simulink model "HIL5DOF_Speedgoat"  (R2026a)
settings: Solver=ode3  StopTime=inf  FixedStep=1/20000
values from neighbouring files (symbols this model uses):
  ems =     [ems11.mat]
  hems =     [Datos_Para_Control_Preciso.mat]
undefined symbols (not defined in the file or in its folder): hems_direct_F_table_H10, hems_direct_gap_bp_H10, hems_direct_I_bp_H10, IO316, IO3xx, m, magnitude, Pull, pull, up, x0, xguid_12, xguid_34, xguid_56, xlev_12, xlev_34, ylev_13, ylev_24, zguid
libraries: speedgoatlib_IO110 x2, aerolibobsolete x1, speedgoatlib_fpga_pwm x1, speedgoatlib_fpga x1
(part 1 of 2)
settings Model: Creator=Mutti  LastModifiedBy=Mutti
settings SolverCC: ConcurrentTasks=on  PositivePriorityOrder=on
settings OptimizationCC: OptimizeBlockIOStorage=off
settings DebuggingCC: TasksWithSamePriorityMsg=none
settings HardwareCC: ProdBitPerLong=64.0  ProdHWDeviceType=Intel->x86-64 (Linux 64)
settings RTWCC: SystemTargetFile=speedgoat.tlc  TemplateMakefile=slrealtime_default_tmf  Toolchain=Simulink Real-Time Toolchain  BuildConfiguration=Faster Runs  TargetLang=C++  Description=Speedgoat Real-Time Target Machine
settings SimulinkRealTimeTargetCC: SLRTFileLogMaxRuns=1.0  TargetLangStandard=C++11 (ISO)  MultiwordLength=2048.0  MATLABClassNameForMDSCustomization=Simulink.SoftwareTarget.GRTCustomization

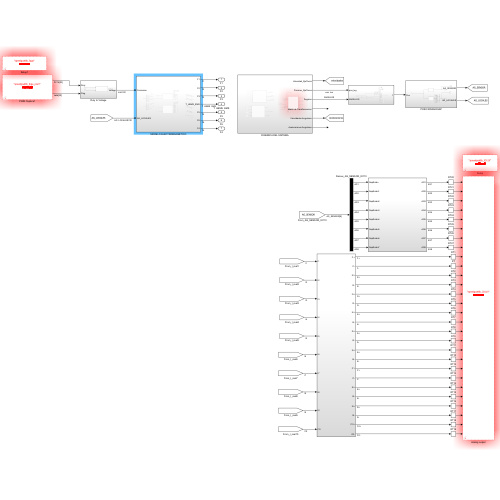
[thumbnail: Simulink's stored preview of the top-level diagram]
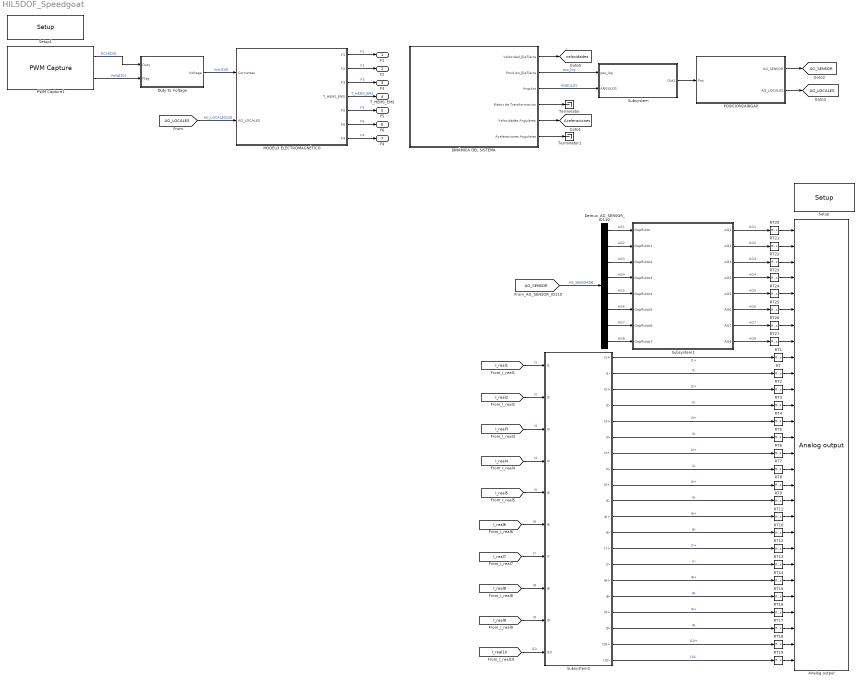
== system HIL5DOF_Speedgoat ==
  Analog output : speedgoatlib_IO110/Analog output  id=1  ts=1/2000  channels=[1,2,3,4,5,6,7,8,9,10,11,12,13,14,15,16,17,18,19,20,21,22,23,24,25,26,27,28]  range=[4,4,4,4,4,4,4,4,4,4,4,4,4,4,4,4,4,4,4,4,4,4,4,4,4,4,4,4,4,4,4,4]  pciSlot=-1  init=[0,0,0,0,0,0,0,0,0,0,0,0,0,0,0,0,0,0,0,0,0,0,0,0,0,0,0,0]  reset=[1,1,1,1,1,1,1,1,1,1,1,1,1,1,1,1,1,1,1,1,1,1,1,1,1,1,1,1]
      settings: SourceProductName=IO110
  DINÁMICA DEL SISTEMA : Subsystem
  Demux_AG_SENSOR_IO110 : Demux  Outputs=8
  Duty to Voltage : Subsystem
  MODELO ELECTROMAGNÉTICO : Subsystem
  POSICION2AIRGAP : Subsystem
  PWM Capture1 : speedgoatlib_fpga_pwm/PWM Capture  id=1  chan=[1:20]  ts=1/1000  captureMode=High transitions triggered  bit_width_cap=24  captureTimeout_si=0.5e-3  captureTimeout_eff=[500e-6]  debounce_si=10e-6  debounce_eff=[10e-6]  showHighDuration=off  showLowDuration=off  showPeriod=off  showDC16=on  showDC8=off  showTOn=off  showTOff=off  showValidData=on
      settings: SourceProductName=PWM
  RT{,1..19} (20 alike) : RateTransition  OutPortSampleTime=5e-05
  RT{20..27} (8 alike) : RateTransition  OutPortSampleTime=1/7500
  Setup : speedgoatlib_IO110/Setup  group=Module setup  id=1  daChannel=[1:28]  daInitValue=zeros(1,28)  daReset=[1]  pciSlot=-1  daRange00=-10V .. +10V  daRange01=-10V .. +10V  daRange02=-10V .. +10V  daRange03=-10V .. +10V  daTSD0=off  daClamp0=on  daRange10=-10V .. +10V  daRange11=-10V .. +10V  daRange12=-10V .. +10V  daRange13=-10V .. +10V  daTSD1=off  daClamp1=on  daRange20=-10V .. +10V  daRange21=-10V .. +10V  daRange22=-10V .. +10V  daRange23=-10V .. +10V  daTSD2=off  daClamp2=on  daRange30=-10V .. +10V  daRange31=-10V .. +10V  daRange32=-10V .. +10V  daRange33=-10V .. +10V  daTSD3=off  daClamp3=on  daRange40=-10V .. +10V  daRange41=-10V .. +10V  daRange42=-10V .. +10V  daRange43=-10V .. +10V  daTSD4=off  daClamp4=on  daRange50=-10V .. +10V  daRange51=-10V .. +10V  daRange52=-10V .. +10V  daRange53=-10V .. +10V  daTSD5=off  daClamp5=on  daRange60=-10V .. +10V  daRange61=-10V .. +10V  daRange62=-10V .. +10V  daRange63=-10V .. +10V  daTSD6=off  daClamp6=on  daRange70=-10V .. +10V  daRange71=-10V .. +10V  daRange72=-10V .. +10V  daRange73=-10V .. +10V  daTSD7=off  daClamp7=on
      settings: SourceProductName=IO110
  Setup1 : speedgoatlib_fpga/Setup/Setup  board=IO316-100k  id=1  pciSlot=-1  device_id=1  bitstreamFilePath=C:\Users\Mutti\Documents\Hyperloop\SpeedGoat\speedgoat_IO316_100k_21_CI_02826_v2\  bitstreamFile=speedgoat_IO316_100k_21_CI_02826_v2.mat  fpgaFreq=[75000000 100000000]  enableDma=off  rearEnb_1=on  rearIO_1=IO3xx-21  rearEnb_2=off  rearIO_2=None  ProgSpiFlash=off  ProgBPIFlash=off  useFpgaDmaController=off  dmaTrigDropdown=Model Step  dmaTrigSelect=0  dmaStopOnOverload=on  dmaModeSequential=on  dmaModeParallel=off  PullRPort15=pull-up 3.3V  PullRPort31=pull-up 3.3V  PullRPort47=pull-up 3.3V  PullRPort63=pull-up 3.3V  diffLineTermination_1=on  diffLineTermination_2=on  diffLineTermination_3=on  diffLineTermination_4=on  diffLineTermination_5=on  diffLineTermination_6=on  diffLineTermination_7=on  diffLineTermination_8=on  diffLineTermination_9=on  diffLineTermination_10=on  diffLineTermination_11=on  diffLineTermination_12=on  diffLineTermination_13=on  diffLineTermination_14=on  diffLineTermination_15=on  diffLineTermination_16=on  diffLineTermination_17=on  diffLineTermination_18=on  diffLineTermination_19=on  diffLineTermination_20=on  diffLineTermination_21=on  diffLineTermination_22=on  diffLineTermination_23=on  diffLineTermination_24=on  diffLineTermination_25=on  diffLineTermination_26=on  diffLineTermination_27=on  diffLineTermination_28=on  diffLineTermination_29=on  diffLineTermination_30=on  diffLineTermination_31=on  diffLineTermination_32=on  ioVoltageDropDown1=3.3V  pullResistorDropDown1_1=Pull-up  pullResistorDropDown1_2=Pull-up  pullResistorDropDown1_3=Pull-up  pullResistorDropDown1_4=Pull-up  pullResistorDropDown1_5=Pull-up  pullResistorDropDown1_6=Pull-up  pullResistorDropDown1_7=Pull-up  pullResistorDropDown1_8=Pull-up  ttlIsImplementedCheckBox1=off  pullResistorDropDown2=Pull-up  ioVoltageDropDown2=3.3V  ttlIsImplementedCheckBox2=off  pullResistorDropDown3=Pull-up  ioVoltageDropDown3=3.3V  ttlIsImplementedCheckBox3=off  pullResistorDropDown4=Pull-up  ioVoltageDropDown4=3.3V  ttlIsImplementedCheckBox4=off  pullResistorDropDown5=Pull-up  ioVoltageDropDown5=3.3V  ttlIsImplementedCheckBox5=off  pullResistorDropDown6=Pull-up  ioVoltageDropDown6=3.3V  ttlIsImplementedCheckBox6=off  pullResistorDropDown7=Pull-up  ioVoltageDropDown7=3.3V  ttlIsImplementedCheckBox7=off  pullResistorDropDown8=Pull-up  ioVoltageDropDown8=3.3V  ttlIsImplementedCheckBox8=off  terminationCheckBox1=off  terminationCheckBox2=off  terminationCheckBox3=off  terminationCheckBox4=off  diffIsImplementedCheckBox1=off  terminationCheckBox5=off  terminationCheckBox6=off  terminationCheckBox7=off  terminationCheckBox8=off  diffIsImplementedCheckBox2=off  terminationCheckBox9=off  terminationCheckBox10=off  terminationCheckBox11=off  terminationCheckBox12=off  diffIsImplementedCheckBox3=off  terminationCheckBox13=off  terminationCheckBox14=off  terminationCheckBox15=off  terminationCheckBox16=off  diffIsImplementedCheckBox4=off  terminationCheckBox17=off  terminationCheckBox18=off  terminationCheckBox19=off  terminationCheckBox20=off  diffIsImplementedCheckBox5=off  terminationCheckBox21=off  terminationCheckBox22=off  terminationCheckBox23=off  terminationCheckBox24=off  diffIsImplementedCheckBox6=off  terminationCheckBox25=off  terminationCheckBox26=off  terminationCheckBox27=off  terminationCheckBox28=off  diffIsImplementedCheckBox7=off  terminationCheckBox29=off  terminationCheckBox30=off  terminationCheckBox31=off  terminationCheckBox32=off  diffIsImplementedCheckBox8=off  PullRPort0_1=pull-up  VioPort0_1=3.3V  PullRPort1_1=pull-up  VioPort1_1=3.3V  PullRPort2_1=pull-up  VioPort2_1=3.3V  PullRPort3_1=pull-up  VioPort3_1=3.3V  PullRPort4_1=pull-up  VioPort4_1=3.3V  PullRPort5_1=pull-up  VioPort5_1=3.3V  PullRPort6_1=pull-up  VioPort6_1=3.3V  diffLineTermination_rear1_1=on  diffLineTermination_rear1_2=on  diffLineTermination_rear1_3=on  diffLineTermination_rear1_4=on  diffLineTermination_rear1_5=on  diffLineTermination_rear1_6=on  diffLineTermination_rear1_7=on  diffLineTermination_rear1_8=on  PullRPort0_2=pull-up  VioPort0_2=3.3V  PullRPort1_2=pull-up  VioPort1_2=3.3V  PullRPort2_2=pull-up  VioPort2_2=3.3V  PullRPort3_2=pull-up  VioPort3_2=3.3V  PullRPort4_2=pull-up  VioPort4_2=3.3V  PullRPort5_2=pull-up  VioPort5_2=3.3V  PullRPort6_2=pull-up  VioPort6_2=3.3V  diffLineTermination_rear2_1=on  diffLineTermination_rear2_2=on  diffLineTermination_rear2_3=on  diffLineTermination_rear2_4=on  diffLineTermination_rear2_5=on  diffLineTermination_rear2_6=on  diffLineTermination_rear2_7=on  diffLineTermination_rear2_8=on
      settings: SourceProductName=IO3xx
  Subsystem : Subsystem
  Subsystem1 : Subsystem
  Subsystem2 : Subsystem
  Terminator : Terminator
  Terminator1 : Terminator
  F1 : Outport
  F2 : Outport  Port=2
  F3 : Outport  Port=3
  T_HEMS_EMS : Outport  Port=4
  F5 : Outport  Port=5
  F6 : Outport  Port=6
  F4 : Outport  Port=7
  tag scope: AG_LOCALES=global, AG_SENSOR=global, Aceleraciones=global, velocidades=global
  wires:
  POSICION2AIRGAP/1(AG_SENSOR) -> [AG_SENSOR]
  POSICION2AIRGAP/2(AG_LOCALES) -> [AG_LOCALES]
  DINÁMICA DEL SISTEMA/4(Matriz de Transformacion) -> Terminator/1
  DINÁMICA DEL SISTEMA/6(Aceleraciones Angulares) -> Terminator1/1
  DINÁMICA DEL SISTEMA/1(Velocidad_EjeTierra) -> [velocidades]
  DINÁMICA DEL SISTEMA/5(Velocidades Angulares) -> [Aceleraciones]
  PWM Capture1/1 -> Duty to Voltage/1(Duty)  "DC16[20]"
  PWM Capture1/2 -> Duty to Voltage/2(Flag)  "Valid[20]"
  Duty to Voltage/1(Voltage) -> MODELO ELECTROMAGNÉTICO/1(Corrientes)  "Vctrl[10]"
  [AG_SENSOR] -> Demux_AG_SENSOR_IO110/1  "AG_SENSOR[8]"
  Demux_AG_SENSOR_IO110/1 -> Subsystem1/1(GapRuido)  "AG1"
  Subsystem1/1(AG1) -> RT20/1  "AG1"
  Demux_AG_SENSOR_IO110/2 -> Subsystem1/2(GapRuido1)  "AG2"
  Subsystem1/2(AG2) -> RT21/1  "AG2"
  Demux_AG_SENSOR_IO110/3 -> Subsystem1/3(GapRuido2)  "AG3"
  Subsystem1/3(AG3) -> RT22/1  "AG3"
  Demux_AG_SENSOR_IO110/4 -> Subsystem1/4(GapRuido3)  "AG4"
  Subsystem1/4(AG4) -> RT23/1  "AG4"
  Demux_AG_SENSOR_IO110/5 -> Subsystem1/5(GapRuido4)  "AG5"
  Subsystem1/5(AG5) -> RT24/1  "AG5"
  Demux_AG_SENSOR_IO110/6 -> Subsystem1/6(GapRuido5)  "AG6"
  Subsystem1/6(AG6) -> RT25/1  "AG6"
  Demux_AG_SENSOR_IO110/7 -> Subsystem1/7(GapRuido6)  "AG7"
  Subsystem1/7(AG7) -> RT26/1  "AG7"
  Demux_AG_SENSOR_IO110/8 -> Subsystem1/8(GapRuido7)  "AG8"
  Subsystem1/8(AG8) -> RT27/1  "AG8"
  [I_real1] -> Subsystem2/1(I1)  "I1"
  [I_real2] -> Subsystem2/2(I2)  "I2"
  [I_real3] -> Subsystem2/3(I3)  "I3"
  [I_real4] -> Subsystem2/4(I4)  "I4"
  [I_real5] -> Subsystem2/5(I5)  "I5"
  [I_real6] -> Subsystem2/6(I6)  "I6"
  [I_real7] -> Subsystem2/7(I7)  "I7"
  [I_real8] -> Subsystem2/8(I8)  "I8"
  [I_real9] -> Subsystem2/9(I9)  "I9"
  [I_real10] -> Subsystem2/10(I10)  "I10"
  Subsystem2/1(I1+) -> RT1/1  "I1+"
  Subsystem2/2(I1-) -> RT/1  "I1-"
  Subsystem2/3(I2+) -> RT2/1  "I2+"
  Subsystem2/4(I2-) -> RT3/1  "I2-"
  Subsystem2/5(I3+) -> RT4/1  "I3+"
  Subsystem2/6(I3-) -> RT5/1  "I3-"
  Subsystem2/7(I4+) -> RT6/1  "I4+"
  Subsystem2/8(I4-) -> RT7/1  "I4-"
  Subsystem2/9(I5+) -> RT8/1  "I5+"
  Subsystem2/10(I5-) -> RT9/1  "I5-"
  Subsystem2/11(I6+) -> RT11/1  "I6+"
  Subsystem2/12(I6-) -> RT10/1  "I6-"
  Subsystem2/13(I7+) -> RT12/1  "I7+"
  Subsystem2/14(I7-) -> RT13/1  "I7-"
  Subsystem2/15(I8+) -> RT14/1  "I8+"
  Subsystem2/16(I8-) -> RT15/1  "I8-"
  Subsystem2/17(I9+) -> RT16/1  "I9+"
  Subsystem2/18(I9-) -> RT17/1  "I9-"
  Subsystem2/19(I10+) -> RT18/1  "I10+"
  Subsystem2/20(I10-) -> RT19/1  "I10-"
  [AG_LOCALES] -> MODELO ELECTROMAGNÉTICO/2(AG_LOCALES)  "AG_LOCALES[10]"
  MODELO ELECTROMAGNÉTICO/1(F1) -> F1/1  "F1"
  MODELO ELECTROMAGNÉTICO/2(F2) -> F2/1  "F2"
  MODELO ELECTROMAGNÉTICO/3(F3) -> F3/1  "F3"
  MODELO ELECTROMAGNÉTICO/4(T_HEMS_EMS) -> T_HEMS_EMS/1  "T_HEMS_EMS"
  MODELO ELECTROMAGNÉTICO/5(F5) -> F5/1  "F5"
  MODELO ELECTROMAGNÉTICO/6(F6) -> F6/1  "F6"
  MODELO ELECTROMAGNÉTICO/7(F4) -> F4/1  "F4"
  RT/1 -> Analog output/10
  RT1/1 -> Analog output/9
  RT2/1 -> Analog output/11
  RT3/1 -> Analog output/12
  RT4/1 -> Analog output/13
  RT5/1 -> Analog output/14
  RT11/1 -> Analog output/19
  RT6/1 -> Analog output/15
  RT7/1 -> Analog output/16
  RT8/1 -> Analog output/17
  RT9/1 -> Analog output/18
  RT10/1 -> Analog output/20
  RT12/1 -> Analog output/21
  RT13/1 -> Analog output/22
  RT14/1 -> Analog output/23
  RT15/1 -> Analog output/24
  RT16/1 -> Analog output/25
  RT17/1 -> Analog output/26
  RT18/1 -> Analog output/27
  RT19/1 -> Analog output/28
  RT20/1 -> Analog output/1
  RT21/1 -> Analog output/2
  RT22/1 -> Analog output/3
  RT23/1 -> Analog output/4
  RT24/1 -> Analog output/5
  RT25/1 -> Analog output/6
  RT26/1 -> Analog output/7
  RT27/1 -> Analog output/8
  DINÁMICA DEL SISTEMA/2(Posicion_EjeTierra) -> Subsystem/1(pos_log)  "pos_log"
  DINÁMICA DEL SISTEMA/3(Ángulos) -> Subsystem/2(ANGULOS)  "ANGULOS"
  Subsystem/1(Out1) -> POSICION2AIRGAP/1(Pos)

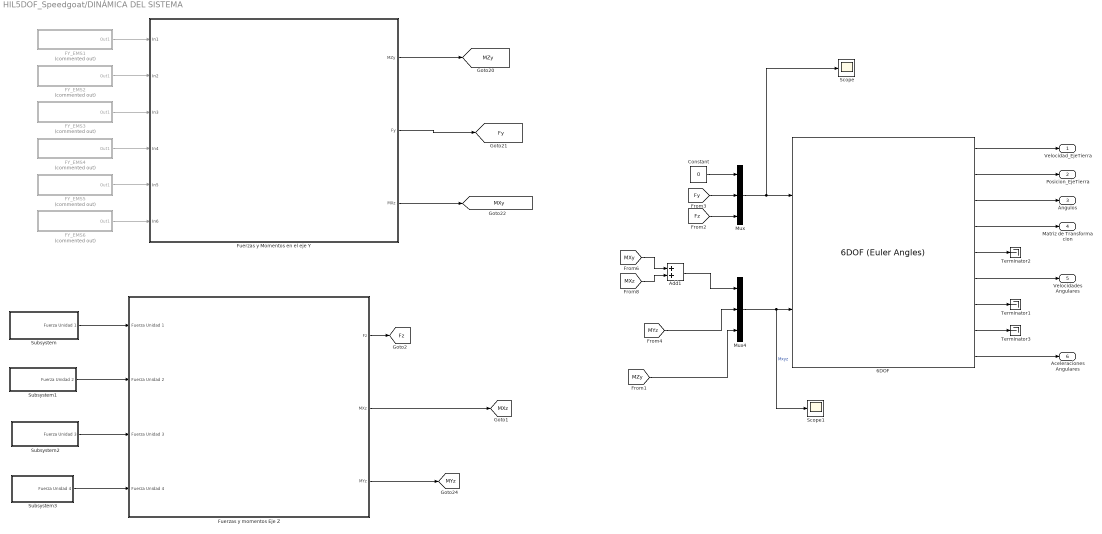
== system HIL5DOF_Speedgoat/DINÁMICA DEL SISTEMA ==
  "6DOF " : aerolibobsolete/6DOF (Euler Angles)  units=Metric (MKS)  mtype=Fixed  rep=Euler Angles  xme_0=[x0 0.000 0.025]  Vm_0=[0 0 0]  eul_0=[0 0 0]  pm_0=[0 0 0]  mass_0=m  mass_e=0.5  mass_f=2.0  inertia=I  inertia_e=eye(3)  inertia_f=2*eye(3)  k_quat=1.0  vre_flag=on  abi_flag=on  aMode=0  xme_statename=''  Vm_statename=''  eul_statename=''  quat_statename=''  pm_statename=''  mass_statename=''
  Add1 : Sum
  Constant : Constant  Value=0
  FY_EMS1 : Subsystem  Commented=on
  FY_EMS2 : Subsystem  Commented=on
  FY_EMS3 : Subsystem  Commented=on
  FY_EMS4 : Subsystem  Commented=on
  FY_EMS5 : Subsystem  Commented=on
  FY_EMS6 : Subsystem  Commented=on
  Fuerzas y Momentos en el eje Y : Subsystem
  Fuerzas y momentos Eje Z : Subsystem
  Mux : Mux  Inputs=3
  Mux4 : Mux  Inputs=3
  Scope : Scope
      settings: ActiveDisplayYMinimum=-6.71767895083E+6  ActiveDisplayYMaximum=4.200096969295E+7
  Scope1 : Scope
      settings: ActiveDisplayYMinimum=-1  ActiveDisplayYMaximum=1  DataLoggingVariableName=ScopeData2
  Subsystem : Subsystem
  Subsystem1 : Subsystem
  Subsystem2 : Subsystem
  Subsystem3 : Subsystem
  Terminator1 : Terminator
  Terminator2 : Terminator
  Terminator3 : Terminator
  Velocidad_EjeTierra : Outport
  Posicion_EjeTierra : Outport  Port=2
  Ángulos : Outport  Port=3
  Matriz de Transformacion : Outport  Port=4
  Velocidades Angulares : Outport  Port=5
  Aceleraciones Angulares : Outport  Port=6
  tag scope: Fy=global, Fz=global, MXy=global, MXz=global, MYz=global, MZy=global
  wires:
  "6DOF "/8 -> Terminator3/1
  "6DOF "/1 -> Velocidad_EjeTierra/1
  "6DOF "/5 -> Terminator2/1
  "6DOF "/4 -> Matriz de Transformacion/1
  "6DOF "/2 -> Posicion_EjeTierra/1
  "6DOF "/3 -> Ángulos/1
  "6DOF "/7 -> Terminator1/1
  "6DOF "/6 -> Velocidades Angulares/1
  [Fy] -> Mux/2
  Mux/1 -> Scope/1, "6DOF "/1
  [Fz] -> Mux/3
  Mux4/1 -> Scope1/1, "6DOF "/2  "Mxyz"
  Constant/1 -> Mux/1
  "6DOF "/9 -> Aceleraciones Angulares/1
  [MZy] -> Mux4/3
  [MXz] -> Add1/2
  [MXy] -> Add1/1
  Fuerzas y momentos Eje Z/1(Fz) -> [Fz]
  Add1/1 -> Mux4/1
  [MYz] -> Mux4/2
  Fuerzas y Momentos en el eje Y/2(Fy) -> [Fy]
  Fuerzas y momentos Eje Z/2(MXz) -> [MXz]
  Fuerzas y momentos Eje Z/3(MYz) -> [MYz]
  Fuerzas y Momentos en el eje Y/3(MXz) -> [MXy]
  Fuerzas y Momentos en el eje Y/1(MZy) -> [MZy]
  FY_EMS1/1(Out1) -> Fuerzas y Momentos en el eje Y/1(In1)
  FY_EMS6/1(Out1) -> Fuerzas y Momentos en el eje Y/6(In6)
  FY_EMS5/1(Out1) -> Fuerzas y Momentos en el eje Y/5(In5)
  FY_EMS4/1(Out1) -> Fuerzas y Momentos en el eje Y/4(In4)
  FY_EMS3/1(Out1) -> Fuerzas y Momentos en el eje Y/3(In3)
  FY_EMS2/1(Out1) -> Fuerzas y Momentos en el eje Y/2(In2)
  Subsystem3/1(Fuerza Unidad 4) -> Fuerzas y momentos Eje Z/4(Fuerza Unidad 4)
  Subsystem/1(Fuerza Unidad 1) -> Fuerzas y momentos Eje Z/1(Fuerza Unidad 1)
  Subsystem1/1(Fuerza Unidad 2) -> Fuerzas y momentos Eje Z/2(Fuerza Unidad 2)
  Subsystem2/1(Fuerza Unidad 3) -> Fuerzas y momentos Eje Z/3(Fuerza Unidad 3)

== system HIL5DOF_Speedgoat/Duty to Voltage ==
  Duty : Inport
  Flag : Inport  Port=2
  PWM pairs to Vctrl : MATLAB Function  TreatAsAtomicUnit=on
  Voltage : Outport
  wires:
  Duty/1 -> PWM pairs to Vctrl/1(Duty)
  Flag/1 -> PWM pairs to Vctrl/2(Flag)
  PWM pairs to Vctrl/1(Voltage) -> Voltage/1

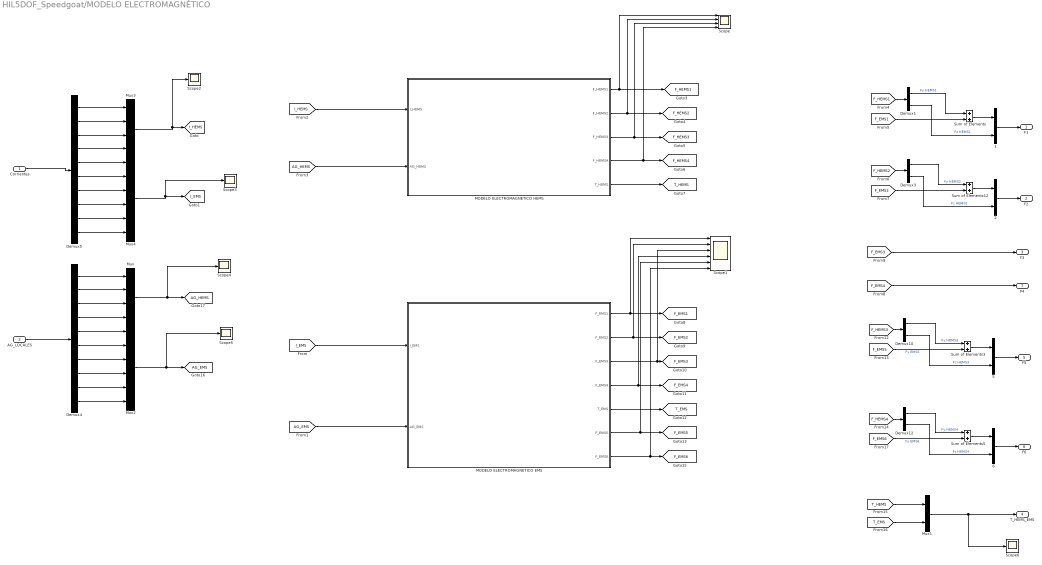
== system HIL5DOF_Speedgoat/MODELO ELECTROMAGNÉTICO ==
  Corrientes : Inport
  AG_LOCALES : Inport  Port=2
  {1..2,5..6} (4 alike) : Mux  Inputs=2
  Demux{1,3,10,12} (4 alike) : Demux  Outputs=2
  Demux4 : Demux  Outputs=10
  Demux5 : Demux  Outputs=10
  MODELO ELECTROMAGNETICO EMS : Subsystem
  MODELO ELECTROMAGNETICO HEMS : Subsystem
  Mux : Mux
  Mux1 : Mux  Inputs=2
  Mux2 : Mux  Inputs=6
  Mux3 : Mux
  Mux4 : Mux  Inputs=6
  Scope : Scope  NumInputPorts=4
      settings: ActiveDisplayYMinimum=225.21547346710162  ActiveDisplayYMaximum=548.6247825703233
  Scope1 : Scope  NumInputPorts=6
      settings: ActiveDisplayYMinimum=-3.137221535142E+7  ActiveDisplayYMaximum=2.1564141928831E+8  DataLoggingVariableName=ScopeData2
  Scope{2..6} (5 alike) : Scope
      Scope2 settings: ActiveDisplayYMinimum=-16.47415  ActiveDisplayYMaximum=23.87015
      Scope3 settings: ActiveDisplayYMinimum=-6.2499999999999982  ActiveDisplayYMaximum=56.25  DataLoggingVariableName=ScopeData2
      Scope4 settings: DataLoggingVariableName=ScopeData3
      Scope5 settings: DataLoggingVariableName=ScopeData4
      Scope6 settings: ActiveDisplayYMinimum=39.93449  ActiveDisplayYMaximum=40.58956  DataLoggingVariableName=ScopeData2
  Sum of Elements{,3,5,12} (4 alike) : Sum
  F1 : Outport
  F2 : Outport  Port=2
  F3 : Outport  Port=3
  T_HEMS_EMS : Outport  Port=4
  F5 : Outport  Port=5
  F6 : Outport  Port=6
  F4 : Outport  Port=7
  tag scope: AG_EMS=global, AG_HEMS=global, F_EMS1=global, F_EMS2=global, F_EMS3=global, F_EMS4=global, F_EMS5=global, F_EMS6=global, F_HEMS1=global, F_HEMS2=global, F_HEMS3=global, F_HEMS4=global, I_EMS=global, I_HEMS=global, T_EMS=global, T_HEMS=global
  wires:
  [I_HEMS] -> MODELO ELECTROMAGNETICO HEMS/1(I_HEMS)
  MODELO ELECTROMAGNETICO HEMS/3(F_HEMS3) -> Scope/3, [F_HEMS3]
  MODELO ELECTROMAGNETICO EMS/5(T_EMS) -> [T_EMS]
  [F_EMS2] -> Sum of Elements12/2
  [F_EMS6] -> Sum of Elements5/2  "Fy EMS6"
  MODELO ELECTROMAGNETICO EMS/3(F_EMS3) -> Scope1/3, [F_EMS3]
  MODELO ELECTROMAGNETICO EMS/6(F_EMS5) -> Scope1/5, [F_EMS5]
  MODELO ELECTROMAGNETICO EMS/1(F_EMS1) -> Scope1/1, [F_EMS1]
  [AG_HEMS] -> MODELO ELECTROMAGNETICO HEMS/2(AG_HEMS)
  Demux12/2 -> 6/2  "Fz HEMS4"
  [I_EMS] -> MODELO ELECTROMAGNETICO EMS/1(I_EMS)
  MODELO ELECTROMAGNETICO HEMS/1(F_HEMS1) -> Scope/1, [F_HEMS1]
  [F_EMS4] -> F4/1
  2/1 -> F2/1
  Demux3/2 -> 2/2  "Fz HEMS2"
  MODELO ELECTROMAGNETICO HEMS/4(F_HEMS4) -> Scope/4, [F_HEMS4]
  MODELO ELECTROMAGNETICO EMS/7(F_EMS6) -> Scope1/6, [F_EMS6]
  Demux1/2 -> 1/2  "Fz HEMS1"
  [T_HEMS] -> Mux1/1
  Sum of Elements/1 -> 1/1
  MODELO ELECTROMAGNETICO HEMS/2(F_HEMS2) -> Scope/2, [F_HEMS2]
  [F_HEMS4] -> Demux12/1
  Sum of Elements12/1 -> 2/1
  5/1 -> F5/1
  [T_EMS] -> Mux1/2
  [F_EMS1] -> Sum of Elements/2
  [F_HEMS2] -> Demux3/1
  Sum of Elements5/1 -> 6/1
  Mux1/1 -> Scope6/1, T_HEMS_EMS/1
  1/1 -> F1/1
  MODELO ELECTROMAGNETICO HEMS/5(T_HEMS) -> [T_HEMS]
  Sum of Elements3/1 -> 5/1
  [F_EMS3] -> F3/1
  [F_HEMS1] -> Demux1/1
  Demux12/1 -> Sum of Elements5/1  "Fy HEMS4"
  [F_EMS5] -> Sum of Elements3/2  "Fy EMS5"
  [F_HEMS3] -> Demux10/1
  [AG_EMS] -> MODELO ELECTROMAGNETICO EMS/2(AG_EMS)
  Demux10/2 -> 5/2  "Fz HEMS3"
  MODELO ELECTROMAGNETICO EMS/4(F_EMS4) -> Scope1/4, [F_EMS4]
  MODELO ELECTROMAGNETICO EMS/2(F_EMS2) -> Scope1/2, [F_EMS2]
  6/1 -> F6/1
  Demux1/1 -> Sum of Elements/1  "Fy HEMS1"
  Demux3/1 -> Sum of Elements12/1  "Fy HEMS2"
  Demux10/1 -> Sum of Elements3/1  "Fy HEMS3"
  AG_LOCALES/1 -> Demux4/1
  Demux4/1 -> Mux/1
  Demux4/2 -> Mux/2
  Demux4/3 -> Mux/3
  Demux4/4 -> Mux/4
  Mux/1 -> Scope4/1, [AG_HEMS]
  Mux2/1 -> Scope5/1, [AG_EMS]
  Demux4/5 -> Mux2/1
  Demux4/10 -> Mux2/6
  Demux4/9 -> Mux2/5
  Demux4/8 -> Mux2/4
  Demux4/7 -> Mux2/3
  Demux4/6 -> Mux2/2
  Demux5/6 -> Mux4/2
  Demux5/7 -> Mux4/3
  Demux5/8 -> Mux4/4
  Demux5/9 -> Mux4/5
  Demux5/10 -> Mux4/6
  Demux5/5 -> Mux4/1
  Mux4/1 -> Scope3/1, [I_EMS]
  Mux3/1 -> Scope2/1, [I_HEMS]
  Demux5/4 -> Mux3/4
  Demux5/3 -> Mux3/3
  Demux5/2 -> Mux3/2
  Demux5/1 -> Mux3/1
  Corrientes/1 -> Demux5/1

== system HIL5DOF_Speedgoat/POSICION2AIRGAP ==
  Pos : Inport
  Demux8 : Demux  Outputs=10
  Mux5 : Mux  Inputs=6
  Mux6 : Mux
  Mux7 : Mux  Inputs=2
  Pos2Airgap_AG_LOCALES : Subsystem
  Pos2Airgap_SENSOR : Subsystem
  Scope1 : Scope
      settings: ActiveDisplayYMinimum=0.0027172435687609548  ActiveDisplayYMaximum=0.025639307881151412  DataLoggingVariableName=ScopeData10
  Scope3 : Scope
      settings: ActiveDisplayYMinimum=-0.049037976197916368  ActiveDisplayYMaximum=0.44139914576247047  DataLoggingVariableName=ScopeData9
  AG_SENSOR : Outport
  AG_LOCALES : Outport  Port=2
  wires:
  Pos2Airgap_SENSOR/1(y) -> Scope3/1, AG_SENSOR/1
  Demux8/8 -> Mux5/4
  Pos2Airgap_AG_LOCALES/1(y) -> Demux8/1
  Demux8/7 -> Mux5/3
  Pos/1 -> Pos2Airgap_SENSOR/1(Pos), Pos2Airgap_AG_LOCALES/1(Pos)
  Mux6/1 -> Mux7/1
  Demux8/9 -> Mux5/5
  Demux8/6 -> Mux5/2
  Mux5/1 -> Mux7/2
  Demux8/3 -> Mux6/3
  Mux7/1 -> Scope1/1, AG_LOCALES/1
  Demux8/4 -> Mux6/4
  Demux8/2 -> Mux6/2
  Demux8/1 -> Mux6/1
  Demux8/10 -> Mux5/6
  Demux8/5 -> Mux5/1

== system HIL5DOF_Speedgoat/Subsystem ==
  pos_log : Inport
  ANGULOS : Inport  Port=2
  Demux : Demux  Outputs=3
  Demux1 : Demux  Outputs=3
  Mux : Mux  Inputs=5
  Mux2 : Mux  Inputs=3
  Saturation1 : Saturate  UpperLimit=0.2  LowerLimit=-0.2
  Saturation2 : Saturate  UpperLimit=0.2  LowerLimit=-0.2
  Saturation3 : Saturate  UpperLimit=0.2  LowerLimit=-0.2
  Saturation4 : Saturate  UpperLimit=0.1  LowerLimit=-0.1
  Saturation5 : Saturate  UpperLimit=0.025  LowerLimit=0.004
  Scope3 : Scope  NumInputPorts=3
      settings: ActiveDisplayYMinimum=0.014784014735112087  ActiveDisplayYMaximum=0.026135109473876435  DataLoggingVariableName=ScopeData12
  Terminator2 : Terminator
  Out1 : Outport
  tag scope: Z=global, angulox=global, anguloy=global, anguloz=global, y_out=global
  wires:
  Mux/1 -> Out1/1
  Saturation2/1 -> Mux2/3, Mux/5, [anguloz]  "ang z"
  Saturation5/1 -> Scope3/2, Mux/2  "z"
  Saturation1/1 -> Mux2/2, Mux/4, [anguloy]  "ang y"
  Demux1/1 -> Saturation3/1
  Demux1/3 -> Saturation2/1
  Demux/1 -> Terminator2/1
  Mux2/1 -> Scope3/3
  Demux/3 -> Saturation5/1, [Z]  "z"
  Saturation3/1 -> [angulox], Mux/3, Mux2/1  "ang x"
  Demux1/2 -> Saturation1/1
  Demux/2 -> [y_out], Saturation4/1  "y"
  Saturation4/1 -> Scope3/1, Mux/1  "y"
  pos_log/1 -> Demux/1
  ANGULOS/1 -> Demux1/1

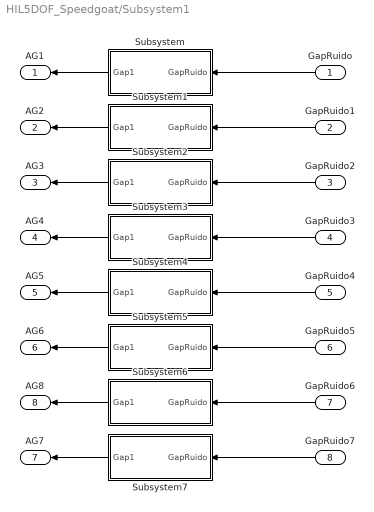
== system HIL5DOF_Speedgoat/Subsystem1 ==
  GapRuido : Inport
  GapRuido1 : Inport  Port=2
  GapRuido2 : Inport  Port=3
  GapRuido3 : Inport  Port=4
  GapRuido4 : Inport  Port=5
  GapRuido5 : Inport  Port=6
  GapRuido6 : Inport  Port=7
  GapRuido7 : Inport  Port=8
  Subsystem : Subsystem
  Subsystem1 : Subsystem
  Subsystem2 : Subsystem
  Subsystem3 : Subsystem
  Subsystem4 : Subsystem
  Subsystem5 : Subsystem
  Subsystem6 : Subsystem
  Subsystem7 : Subsystem
  AG1 : Outport
  AG2 : Outport  Port=2
  AG3 : Outport  Port=3
  AG4 : Outport  Port=4
  AG5 : Outport  Port=5
  AG6 : Outport  Port=6
  AG7 : Outport  Port=7
  AG8 : Outport  Port=8
  wires:
  Subsystem/1(Gap1) -> AG1/1
  Subsystem3/1(Gap1) -> AG4/1
  Subsystem1/1(Gap1) -> AG2/1
  Subsystem2/1(Gap1) -> AG3/1
  Subsystem4/1(Gap1) -> AG5/1
  Subsystem5/1(Gap1) -> AG6/1
  Subsystem7/1(Gap1) -> AG7/1
  Subsystem6/1(Gap1) -> AG8/1
  GapRuido/1 -> Subsystem/1(GapRuido)
  GapRuido1/1 -> Subsystem1/1(GapRuido)
  GapRuido2/1 -> Subsystem2/1(GapRuido)
  GapRuido3/1 -> Subsystem3/1(GapRuido)
  GapRuido4/1 -> Subsystem4/1(GapRuido)
  GapRuido5/1 -> Subsystem5/1(GapRuido)
  GapRuido6/1 -> Subsystem6/1(GapRuido)
  GapRuido7/1 -> Subsystem7/1(GapRuido)

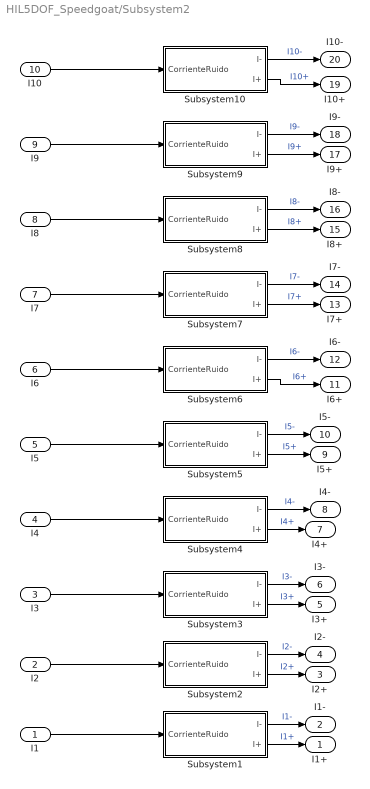
== system HIL5DOF_Speedgoat/Subsystem2 ==
  I1 : Inport
  I2 : Inport  Port=2
  I3 : Inport  Port=3
  I4 : Inport  Port=4
  I5 : Inport  Port=5
  I6 : Inport  Port=6
  I7 : Inport  Port=7
  I8 : Inport  Port=8
  I9 : Inport  Port=9
  I10 : Inport  Port=10
  Subsystem1 : Subsystem
  Subsystem10 : Subsystem
  Subsystem2 : Subsystem
  Subsystem3 : Subsystem
  Subsystem4 : Subsystem
  Subsystem5 : Subsystem
  Subsystem6 : Subsystem
  Subsystem7 : Subsystem
  Subsystem8 : Subsystem
  Subsystem9 : Subsystem
  I1+ : Outport
  I1- : Outport  Port=2
  I2+ : Outport  Port=3
  I2- : Outport  Port=4
  I3+ : Outport  Port=5
  I3- : Outport  Port=6
  I4+ : Outport  Port=7
  I4- : Outport  Port=8
  I5+ : Outport  Port=9
  I5- : Outport  Port=10
  I6+ : Outport  Port=11
  I6- : Outport  Port=12
  I7+ : Outport  Port=13
  I7- : Outport  Port=14
  I8+ : Outport  Port=15
  I8- : Outport  Port=16
  I9+ : Outport  Port=17
  I9- : Outport  Port=18
  I10+ : Outport  Port=19
  I10- : Outport  Port=20
  wires:
  Subsystem1/1(I-) -> I1-/1  "I1-"
  Subsystem1/2(I+) -> I1+/1  "I1+"
  Subsystem2/1(I-) -> I2-/1  "I2-"
  Subsystem2/2(I+) -> I2+/1  "I2+"
  I1/1 -> Subsystem1/1(CorrienteRuido)
  I10/1 -> Subsystem10/1(CorrienteRuido)
  I9/1 -> Subsystem9/1(CorrienteRuido)
  I8/1 -> Subsystem8/1(CorrienteRuido)
  I7/1 -> Subsystem7/1(CorrienteRuido)
  I6/1 -> Subsystem6/1(CorrienteRuido)
  I5/1 -> Subsystem5/1(CorrienteRuido)
  I3/1 -> Subsystem3/1(CorrienteRuido)
  I4/1 -> Subsystem4/1(CorrienteRuido)
  I2/1 -> Subsystem2/1(CorrienteRuido)
  Subsystem3/2(I+) -> I3+/1  "I3+"
  Subsystem3/1(I-) -> I3-/1  "I3-"
  Subsystem4/2(I+) -> I4+/1  "I4+"
  Subsystem4/1(I-) -> I4-/1  "I4-"
  Subsystem5/2(I+) -> I5+/1  "I5+"
  Subsystem5/1(I-) -> I5-/1  "I5-"
  Subsystem6/2(I+) -> I6+/1  "I6+"
  Subsystem6/1(I-) -> I6-/1  "I6-"
  Subsystem7/2(I+) -> I7+/1  "I7+"
  Subsystem7/1(I-) -> I7-/1  "I7-"
  Subsystem8/2(I+) -> I8+/1  "I8+"
  Subsystem8/1(I-) -> I8-/1  "I8-"
  Subsystem9/2(I+) -> I9+/1  "I9+"
  Subsystem9/1(I-) -> I9-/1  "I9-"
  Subsystem10/2(I+) -> I10+/1  "I10+"
  Subsystem10/1(I-) -> I10-/1  "I10-"

== system HIL5DOF_Speedgoat/DINÁMICA DEL SISTEMA/FY_EMS1 ==
  Out1 : Outport
  wires:
  [Fy_EMS1] -> Out1/1

== system HIL5DOF_Speedgoat/DINÁMICA DEL SISTEMA/FY_EMS2 ==
  Out1 : Outport
  wires:
  [Fy_EMS2] -> Out1/1

== system HIL5DOF_Speedgoat/DINÁMICA DEL SISTEMA/FY_EMS3 ==
  Out1 : Outport
  wires:
  [Fy_EMS3] -> Out1/1

== system HIL5DOF_Speedgoat/DINÁMICA DEL SISTEMA/FY_EMS4 ==
  Out1 : Outport
  wires:
  [Fy_EMS4] -> Out1/1

== system HIL5DOF_Speedgoat/DINÁMICA DEL SISTEMA/FY_EMS5 ==
  Out1 : Outport
  wires:
  [Fy_EMS5] -> Out1/1

== system HIL5DOF_Speedgoat/DINÁMICA DEL SISTEMA/FY_EMS6 ==
  Out1 : Outport
  wires:
  [Fy_EMS6] -> Out1/1

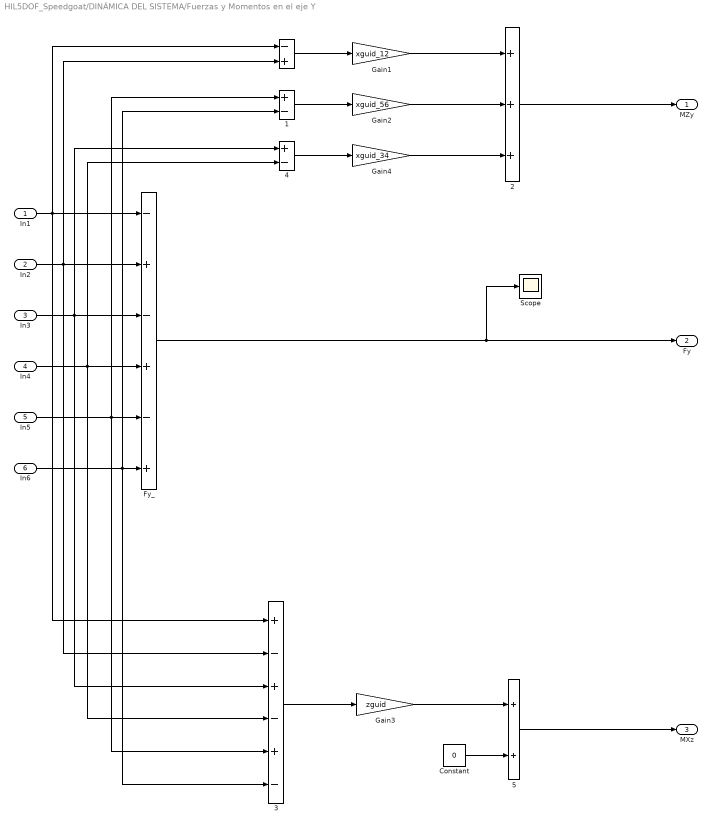
== system HIL5DOF_Speedgoat/DINÁMICA DEL SISTEMA/Fuerzas y Momentos en el eje Y ==
  In1 : Inport
  In2 : Inport  Port=2
  In3 : Inport  Port=3
  In4 : Inport  Port=4
  In5 : Inport  Port=5
  In6 : Inport  Port=6
  " " : Sum  Inputs=-+
  " 1" : Sum  Inputs=+-
  " 2" : Sum  Inputs=+++
  " 3" : Sum  Inputs=+-+-+-
  " 4" : Sum  Inputs=+-
  " 5" : Sum
  Constant : Constant  Value=0
  Fy_ : Sum  Inputs=-+-+-+
  Gain1 : Gain  Gain=xguid_12
  Gain2 : Gain  Gain=xguid_56
  Gain3 : Gain  Gain=zguid
  Gain4 : Gain  Gain=xguid_34
  Scope : Scope
      settings: ActiveDisplayYMinimum=-46.4281  ActiveDisplayYMaximum=9.86806
  MZy : Outport
  Fy : Outport  Port=2
  MXz : Outport  Port=3
  wires:
  " 5"/1 -> MXz/1
  " 3"/1 -> Gain3/1
  In3/1 -> " 4"/1, Fy_/3, " 3"/3
  " 2"/1 -> MZy/1
  " 1"/1 -> Gain2/1
  " "/1 -> Gain1/1
  In4/1 -> " 3"/4, " 4"/2, Fy_/4
  Gain3/1 -> " 5"/1
  Fy_/1 -> Scope/1, Fy/1
  In6/1 -> " 3"/6, " 1"/2, Fy_/6
  In5/1 -> " 3"/5, " 1"/1, Fy_/5
  In2/1 -> " 3"/2, Fy_/2, " "/2
  In1/1 -> " 3"/1, " "/1, Fy_/1
  Constant/1 -> " 5"/2
  Gain1/1 -> " 2"/1
  Gain2/1 -> " 2"/2
  Gain4/1 -> " 2"/3
  " 4"/1 -> Gain4/1

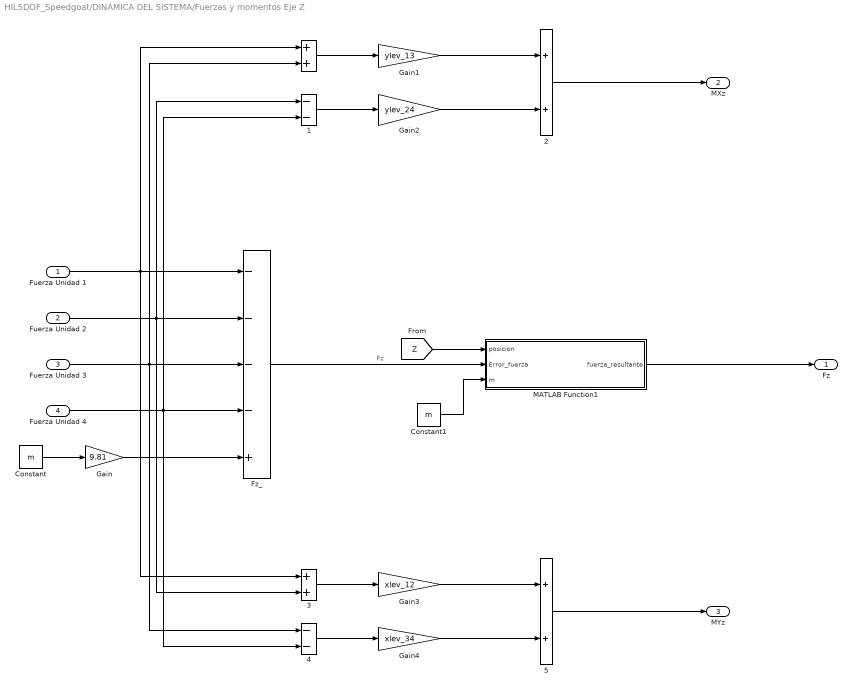
== system HIL5DOF_Speedgoat/DINÁMICA DEL SISTEMA/Fuerzas y momentos Eje Z ==
  Fuerza Unidad 1 : Inport
  Fuerza Unidad 2 : Inport  Port=2
  Fuerza Unidad 3 : Inport  Port=3
  Fuerza Unidad 4 : Inport  Port=4
   {,2..3,5} (4 alike) : Sum
  " 1" : Sum  Inputs=--
  " 4" : Sum  Inputs=--
  Constant : Constant  Value=m
  Constant1 : Constant  Value=m
  Fz_ : Sum  Inputs=----+
  Gain : Gain  Gain=9.81
  Gain1 : Gain  Gain=ylev_13
  Gain2 : Gain  Gain=ylev_24
  Gain3 : Gain  Gain=xlev_12
  Gain4 : Gain  Gain=xlev_34
  MATLAB Function1 : MATLAB Function  TreatAsAtomicUnit=on
  Fz : Outport
  MXz : Outport  Port=2
  MYz : Outport  Port=3
  wires:
  " 4"/1 -> Gain4/1
  " 3"/1 -> Gain3/1
  Fuerza Unidad 3/1 -> " 4"/1, " "/2, Fz_/3
  Fuerza Unidad 1/1 -> " 3"/1, " "/1, Fz_/1
  Fuerza Unidad 2/1 -> Fz_/2, " 3"/2, " 1"/1
  Gain1/1 -> " 2"/1
  " 2"/1 -> MXz/1
  Gain3/1 -> " 5"/1
  Gain4/1 -> " 5"/2
  Gain2/1 -> " 2"/2
  " "/1 -> Gain1/1
  Fuerza Unidad 4/1 -> " 4"/2, " 1"/2, Fz_/4
  " 5"/1 -> MYz/1
  " 1"/1 -> Gain2/1
  Constant/1 -> Gain/1
  Gain/1 -> Fz_/5
  [Z] -> MATLAB Function1/1(posicion)
  Fz_/1 -> MATLAB Function1/2(Error_fuerza)  "Fz"
  MATLAB Function1/1(fuerza_resultante) -> Fz/1
  Constant1/1 -> MATLAB Function1/3(m)

== system HIL5DOF_Speedgoat/DINÁMICA DEL SISTEMA/Subsystem ==
  Fuerza Unidad 1 : Outport
  wires:
  [Fz_HEMS1] -> Fuerza Unidad 1/1

== system HIL5DOF_Speedgoat/DINÁMICA DEL SISTEMA/Subsystem1 ==
  Fuerza Unidad 2 : Outport
  wires:
  [Fz_HEMS2] -> Fuerza Unidad 2/1

== system HIL5DOF_Speedgoat/DINÁMICA DEL SISTEMA/Subsystem2 ==
  Fuerza Unidad 3 : Outport
  wires:
  [Fz_HEMS3] -> Fuerza Unidad 3/1

== system HIL5DOF_Speedgoat/DINÁMICA DEL SISTEMA/Subsystem3 ==
  Fuerza Unidad 4 : Outport
  wires:
  [Fz_HEMS4] -> Fuerza Unidad 4/1

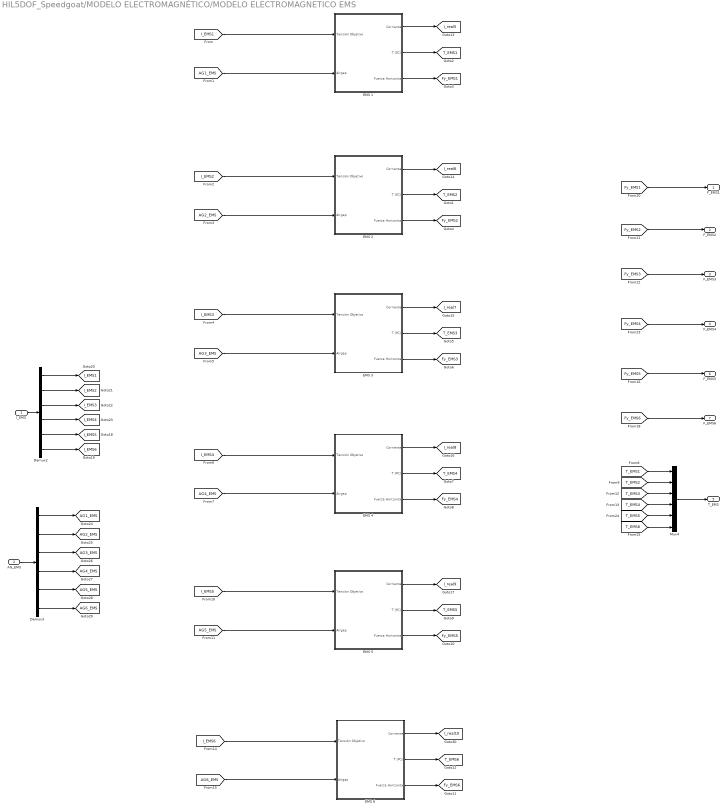
== system HIL5DOF_Speedgoat/MODELO ELECTROMAGNÉTICO/MODELO ELECTROMAGNETICO EMS ==
  I_EMS : Inport
  AG_EMS : Inport  Port=2
  Demux2 : Demux  Outputs=6
  Demux3 : Demux  Outputs=6
  EMS 1 : Subsystem
  EMS 2 : Subsystem
  EMS 3 : Subsystem
  EMS 4 : Subsystem
  EMS 5 : Subsystem
  EMS 6 : Subsystem
  Mux4 : Mux  Inputs=6
  F_EMS1 : Outport
  F_EMS2 : Outport  Port=2
  F_EMS3 : Outport  Port=3
  F_EMS4 : Outport  Port=4
  T_EMS : Outport  Port=5
  F_EMS5 : Outport  Port=6
  F_EMS6 : Outport  Port=7
  tag scope: AG1_EMS=global, AG2_EMS=global, AG3_EMS=global, AG4_EMS=global, AG5_EMS=global, AG6_EMS=global, Fy_EMS1=global, Fy_EMS2=global, Fy_EMS3=global, Fy_EMS4=global, Fy_EMS5=global, Fy_EMS6=global, I_EMS1=global, I_EMS2=global, I_EMS3=global, I_EMS4=global, I_EMS5=global, I_EMS6=global, I_real10=global, I_real5=global, I_real6=global, I_real7=global, I_real8=global, I_real9=global, T_EMS1=global, T_EMS2=global, T_EMS3=global, T_EMS4=global, T_EMS5=global, T_EMS6=global
  wires:
  EMS 1/2(T [ºC]) -> [T_EMS1]
  [T_EMS2] -> Mux4/2
  [Fy_EMS2] -> F_EMS2/1
  [Fy_EMS4] -> F_EMS4/1
  [AG1_EMS] -> EMS 1/2(Airgap)
  EMS 1/3(Fuerza Horizontal) -> [Fy_EMS1]
  Mux4/1 -> T_EMS/1
  [T_EMS3] -> Mux4/3
  [I_EMS1] -> EMS 1/1(Tensión Objetivo)
  [Fy_EMS1] -> F_EMS1/1
  [T_EMS1] -> Mux4/1
  [T_EMS4] -> Mux4/4
  [Fy_EMS3] -> F_EMS3/1
  Demux2/2 -> [I_EMS2]
  AG_EMS/1 -> Demux3/1
  Demux3/2 -> [AG2_EMS]
  Demux2/3 -> [I_EMS3]
  Demux2/1 -> [I_EMS1]
  Demux3/1 -> [AG1_EMS]
  Demux2/4 -> [I_EMS4]
  Demux3/4 -> [AG4_EMS]
  I_EMS/1 -> Demux2/1
  Demux3/3 -> [AG3_EMS]
  [Fy_EMS5] -> F_EMS5/1
  [Fy_EMS6] -> F_EMS6/1
  [T_EMS5] -> Mux4/5
  [T_EMS6] -> Mux4/6
  Demux2/5 -> [I_EMS5]
  Demux2/6 -> [I_EMS6]
  Demux3/5 -> [AG5_EMS]
  Demux3/6 -> [AG6_EMS]
  EMS 2/3(Fuerza Horizontal) -> [Fy_EMS2]
  [AG2_EMS] -> EMS 2/2(Airgap)
  EMS 2/2(T [ºC]) -> [T_EMS2]
  EMS 3/2(T [ºC]) -> [T_EMS3]
  [AG3_EMS] -> EMS 3/2(Airgap)
  EMS 3/3(Fuerza Horizontal) -> [Fy_EMS3]
  [I_EMS4] -> EMS 4/1(Tensión Objetivo)
  EMS 4/3(Fuerza Horizontal) -> [Fy_EMS4]
  [AG4_EMS] -> EMS 4/2(Airgap)
  EMS 4/2(T [ºC]) -> [T_EMS4]
  EMS 5/2(T [ºC]) -> [T_EMS5]
  [AG5_EMS] -> EMS 5/2(Airgap)
  EMS 5/3(Fuerza Horizontal) -> [Fy_EMS5]
  [I_EMS6] -> EMS 6/1(Tensión Objetivo)
  EMS 6/3(Fuerza Horizontal) -> [Fy_EMS6]
  [AG6_EMS] -> EMS 6/2(Airgap)
  EMS 6/2(T [ºC]) -> [T_EMS6]
  EMS 6/1(Corriente) -> [I_real10]
  EMS 1/1(Corriente) -> [I_real5]
  EMS 2/1(Corriente) -> [I_real6]
  EMS 3/1(Corriente) -> [I_real7]
  EMS 4/1(Corriente) -> [I_real8]
  EMS 5/1(Corriente) -> [I_real9]
  [I_EMS3] -> EMS 3/1(Tensión Objetivo)
  [I_EMS5] -> EMS 5/1(Tensión Objetivo)
  [I_EMS2] -> EMS 2/1(Tensión Objetivo)

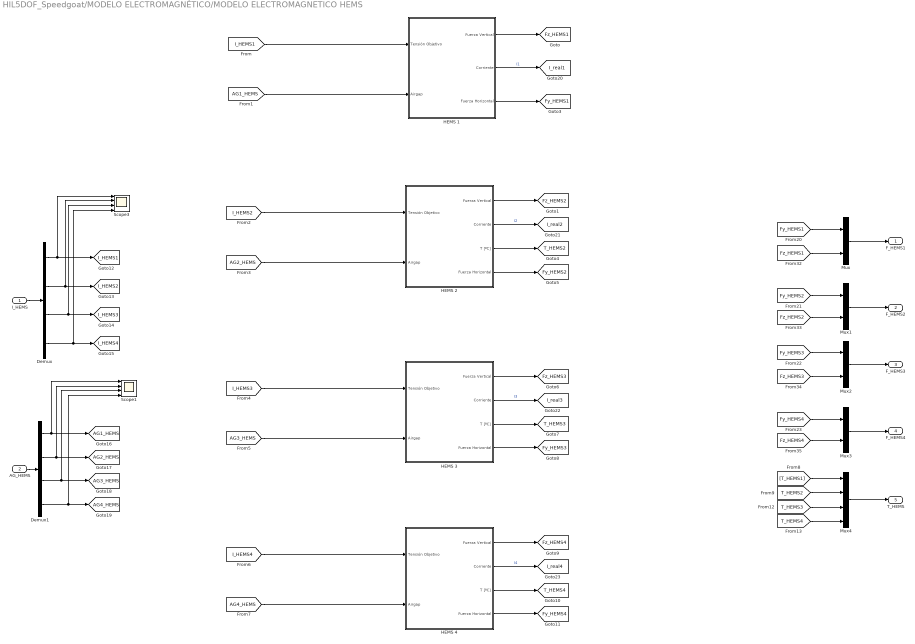
== system HIL5DOF_Speedgoat/MODELO ELECTROMAGNÉTICO/MODELO ELECTROMAGNETICO HEMS ==
  I_HEMS : Inport
  AG_HEMS : Inport  Port=2
  Demux : Demux
  Demux1 : Demux
  HEMS 1 : Subsystem
  HEMS 2 : Subsystem
  HEMS 3 : Subsystem
  HEMS 4 : Subsystem
  Mux{,1..3} (4 alike) : Mux  Inputs=2
  Mux4 : Mux
  Scope1 : Scope  NumInputPorts=4
      settings: ActiveDisplayYMinimum=-1  ActiveDisplayYMaximum=1  DataLoggingVariableName=ScopeData6
  Scope3 : Scope  NumInputPorts=4
      settings: ActiveDisplayYMinimum=-1.255420573512E+7  ActiveDisplayYMaximum=1.335448688442E+7  DataLoggingVariableName=ScopeData5
  F_HEMS1 : Outport
  F_HEMS2 : Outport  Port=2
  F_HEMS3 : Outport  Port=3
  F_HEMS4 : Outport  Port=4
  T_HEMS : Outport  Port=5
  tag scope: AG1_HEMS=global, AG2_HEMS=global, AG3_HEMS=global, AG4_HEMS=global, Fy_HEMS1=global, Fy_HEMS2=global, Fy_HEMS3=global, Fy_HEMS4=global, Fz_HEMS1=global, Fz_HEMS2=global, Fz_HEMS3=global, Fz_HEMS4=global, I_HEMS1=global, I_HEMS2=global, I_HEMS3=global, I_HEMS4=global, I_real1=global, I_real2=global, I_real3=global, I_real4=global, T_HEMS2=global, T_HEMS3=global, T_HEMS4=global
  wires:
  Mux2/1 -> F_HEMS3/1
  [Fz_HEMS2] -> Mux1/2
  [I_HEMS4] -> HEMS 4/1(Tensión Objetivo)
  [Fy_HEMS1] -> Mux/1
  I_HEMS/1 -> Demux/1
  [T_HEMS4] -> Mux4/4
  [T_HEMS1] -> Mux4/1
  [I_HEMS3] -> HEMS 3/1(Tensión Objetivo)
  [Fy_HEMS2] -> Mux1/1
  Mux/1 -> F_HEMS1/1
  [I_HEMS2] -> HEMS 2/1(Tensión Objetivo)
  [I_HEMS1] -> HEMS 1/1(Tensión Objetivo)
  [T_HEMS3] -> Mux4/3
  HEMS 1/1(Fuerza Vertical) -> [Fz_HEMS1]
  Mux4/1 -> T_HEMS/1
  [AG3_HEMS] -> HEMS 3/2(Airgap)
  Demux/4 -> Scope3/4, [I_HEMS4]
  Demux1/1 -> Scope1/1, [AG1_HEMS]
  HEMS 4/1(Fuerza Vertical) -> [Fz_HEMS4]
  HEMS 1/3(Fuerza Horizontal) -> [Fy_HEMS1]
  HEMS 3/4(Fuerza Horizontal) -> [Fy_HEMS3]
  [AG1_HEMS] -> HEMS 1/2(Airgap)
  [Fy_HEMS3] -> Mux2/1
  Mux3/1 -> F_HEMS4/1
  [Fz_HEMS3] -> Mux2/2
  Mux1/1 -> F_HEMS2/1
  [T_HEMS2] -> Mux4/2
  [Fz_HEMS4] -> Mux3/2
  HEMS 3/3(T [ºC]) -> [T_HEMS3]
  Demux/1 -> Scope3/1, [I_HEMS1]
  HEMS 3/1(Fuerza Vertical) -> [Fz_HEMS3]
  Demux/2 -> Scope3/2, [I_HEMS2]
  [AG4_HEMS] -> HEMS 4/2(Airgap)
  Demux1/3 -> Scope1/3, [AG3_HEMS]
  [AG2_HEMS] -> HEMS 2/2(Airgap)
  Demux1/4 -> Scope1/4, [AG4_HEMS]
  Demux/3 -> Scope3/3, [I_HEMS3]
  AG_HEMS/1 -> Demux1/1
  Demux1/2 -> Scope1/2, [AG2_HEMS]
  HEMS 4/3(T [ºC]) -> [T_HEMS4]
  HEMS 4/4(Fuerza Horizontal) -> [Fy_HEMS4]
  [Fy_HEMS4] -> Mux3/1
  HEMS 2/1(Fuerza Vertical) -> [Fz_HEMS2]
  HEMS 2/3(T [ºC]) -> [T_HEMS2]
  HEMS 2/4(Fuerza Horizontal) -> [Fy_HEMS2]
  [Fz_HEMS1] -> Mux/2
  HEMS 2/2(Corriente) -> [I_real2]  "I2"
  HEMS 4/2(Corriente) -> [I_real4]  "I4"
  HEMS 3/2(Corriente) -> [I_real3]  "I3"
  HEMS 1/2(Corriente) -> [I_real1]  "I1"

== system HIL5DOF_Speedgoat/POSICION2AIRGAP/Pos2Airgap_AG_LOCALES ==
  Pos : Inport
  Demux2 : Demux  Outputs=5
  MATLAB Function : MATLAB Function  TreatAsAtomicUnit=on
  Mux1 : Mux  Inputs=5
  y : Outport
  wires:
  Demux2/3 -> Mux1/3
  Demux2/2 -> Mux1/2
  Demux2/4 -> Mux1/4
  Mux1/1 -> MATLAB Function/1(posicion)
  Demux2/5 -> Mux1/5
  Demux2/1 -> Mux1/1
  Pos/1 -> Demux2/1
  MATLAB Function/1(airgaps_actuadores) -> y/1

== system HIL5DOF_Speedgoat/POSICION2AIRGAP/Pos2Airgap_SENSOR ==
  Pos : Inport
  Demux2 : Demux  Outputs=5
  MATLAB Function : MATLAB Function  TreatAsAtomicUnit=on
  Mux1 : Mux  Inputs=5
  y : Outport
  wires:
  Pos/1 -> Demux2/1
  Demux2/1 -> Mux1/1
  Demux2/5 -> Mux1/5
  Mux1/1 -> MATLAB Function/1(estados)
  Demux2/4 -> Mux1/4
  Demux2/2 -> Mux1/2
  Demux2/3 -> Mux1/3
  MATLAB Function/1(gaps) -> y/1

== system HIL5DOF_Speedgoat/Subsystem1/Subsystem ==
  GapRuido : Inport
  Gainp : Gain  Gain=3/0.0225
  Sat Pos : Saturate  UpperLimit=3.3  LowerLimit=0
  Gap1 : Outport
  wires:
  Sat Pos/1 -> Gap1/1
  GapRuido/1 -> Gainp/1
  Gainp/1 -> Sat Pos/1

== system HIL5DOF_Speedgoat/Subsystem1/Subsystem1 ==
  GapRuido : Inport
  Gainp : Gain  Gain=3/0.0225
  Sat Pos : Saturate  UpperLimit=3.3  LowerLimit=0
  Gap1 : Outport
  wires:
  Sat Pos/1 -> Gap1/1
  GapRuido/1 -> Gainp/1
  Gainp/1 -> Sat Pos/1

== system HIL5DOF_Speedgoat/Subsystem1/Subsystem2 ==
  GapRuido : Inport
  Gainp : Gain  Gain=3/0.0225
  Sat Pos : Saturate  UpperLimit=3.3  LowerLimit=0
  Gap1 : Outport
  wires:
  Sat Pos/1 -> Gap1/1
  GapRuido/1 -> Gainp/1
  Gainp/1 -> Sat Pos/1

== system HIL5DOF_Speedgoat/Subsystem1/Subsystem3 ==
  GapRuido : Inport
  Gainp : Gain  Gain=3/0.0225
  Sat Pos : Saturate  UpperLimit=3.3  LowerLimit=0
  Gap1 : Outport
  wires:
  Sat Pos/1 -> Gap1/1
  GapRuido/1 -> Gainp/1
  Gainp/1 -> Sat Pos/1

== system HIL5DOF_Speedgoat/Subsystem1/Subsystem4 ==
  GapRuido : Inport
  Gainp : Gain  Gain=3/0.0225
  Sat Pos : Saturate  UpperLimit=3.3  LowerLimit=0
  Gap1 : Outport
  wires:
  Sat Pos/1 -> Gap1/1
  GapRuido/1 -> Gainp/1
  Gainp/1 -> Sat Pos/1

== system HIL5DOF_Speedgoat/Subsystem1/Subsystem5 ==
  GapRuido : Inport
  Gainp : Gain  Gain=3/0.0225
  Sat Pos : Saturate  UpperLimit=3.3  LowerLimit=0
  Gap1 : Outport
  wires:
  Sat Pos/1 -> Gap1/1
  GapRuido/1 -> Gainp/1
  Gainp/1 -> Sat Pos/1

== system HIL5DOF_Speedgoat/Subsystem1/Subsystem6 ==
  GapRuido : Inport
  Gainp : Gain  Gain=3/0.0225
  Sat Pos : Saturate  UpperLimit=3.3  LowerLimit=0
  Gap1 : Outport
  wires:
  Sat Pos/1 -> Gap1/1
  GapRuido/1 -> Gainp/1
  Gainp/1 -> Sat Pos/1

== system HIL5DOF_Speedgoat/Subsystem1/Subsystem7 ==
  GapRuido : Inport
  Gainp : Gain  Gain=3/0.0225
  Sat Pos : Saturate  UpperLimit=3.3  LowerLimit=0
  Gap1 : Outport
  wires:
  Sat Pos/1 -> Gap1/1
  GapRuido/1 -> Gainp/1
  Gainp/1 -> Sat Pos/1

== system HIL5DOF_Speedgoat/Subsystem2/Subsystem1 ==
  CorrienteRuido : Inport
  Constant4 : Constant  Value=1.44
  Constant5 : Constant  Value=5.23
  Gain2 : Gain  Gain=(500/1000000)*41/2
  Gain3 : Gain  Gain=(500/1000000)*41/2
  Gain4 : Gain  Gain=1/1.326
  Sat Cur : Saturate  UpperLimit=3.3  LowerLimit=0
  Sat Cur1 : Saturate  UpperLimit=3.3  LowerLimit=0
  Sum2 : Sum  Inputs=|-+
  Sum3 : Sum  Inputs=|++
  Sum4 : Sum  Inputs=|+-
  I- : Outport
  I+ : Outport  Port=2
  wires:
  Sat Cur/1 -> I-/1
  Sum4/1 -> Gain4/1
  Gain4/1 -> Gain3/1, Gain2/1
  Sat Cur1/1 -> I+/1
  CorrienteRuido/1 -> Sum4/1
  Constant4/1 -> Sum3/2, Sum2/2
  Sum3/1 -> Sat Cur1/1
  Gain2/1 -> Sum2/1
  Sum2/1 -> Sat Cur/1
  Constant5/1 -> Sum4/2
  Gain3/1 -> Sum3/1

== system HIL5DOF_Speedgoat/Subsystem2/Subsystem10 ==
  CorrienteRuido : Inport
  Constant4 : Constant  Value=1.44
  Constant5 : Constant  Value=5.23
  Gain2 : Gain  Gain=(500/1000000)*41/2
  Gain3 : Gain  Gain=(500/1000000)*41/2
  Gain4 : Gain  Gain=1/1.326
  Sat Cur : Saturate  UpperLimit=3.3  LowerLimit=0
  Sat Cur1 : Saturate  UpperLimit=3.3  LowerLimit=0
  Sum2 : Sum  Inputs=|-+
  Sum3 : Sum  Inputs=|++
  Sum4 : Sum  Inputs=|+-
  I- : Outport
  I+ : Outport  Port=2
  wires:
  Sat Cur/1 -> I-/1
  Sum4/1 -> Gain4/1
  Gain4/1 -> Gain3/1, Gain2/1
  Sat Cur1/1 -> I+/1
  CorrienteRuido/1 -> Sum4/1
  Constant4/1 -> Sum3/2, Sum2/2
  Sum3/1 -> Sat Cur1/1
  Gain2/1 -> Sum2/1
  Sum2/1 -> Sat Cur/1
  Constant5/1 -> Sum4/2
  Gain3/1 -> Sum3/1

== system HIL5DOF_Speedgoat/Subsystem2/Subsystem2 ==
  CorrienteRuido : Inport
  Constant4 : Constant  Value=1.44
  Constant5 : Constant  Value=5.23
  Gain2 : Gain  Gain=(500/1000000)*41/2
  Gain3 : Gain  Gain=(500/1000000)*41/2
  Gain4 : Gain  Gain=1/1.326
  Sat Cur : Saturate  UpperLimit=3.3  LowerLimit=0
  Sat Cur1 : Saturate  UpperLimit=3.3  LowerLimit=0
  Sum2 : Sum  Inputs=|-+
  Sum3 : Sum  Inputs=|++
  Sum4 : Sum  Inputs=|+-
  I- : Outport
  I+ : Outport  Port=2
  wires:
  Sat Cur/1 -> I-/1
  Sum4/1 -> Gain4/1
  Gain4/1 -> Gain3/1, Gain2/1
  Sat Cur1/1 -> I+/1
  CorrienteRuido/1 -> Sum4/1
  Constant4/1 -> Sum3/2, Sum2/2
  Sum3/1 -> Sat Cur1/1
  Gain2/1 -> Sum2/1
  Sum2/1 -> Sat Cur/1
  Constant5/1 -> Sum4/2
  Gain3/1 -> Sum3/1

== system HIL5DOF_Speedgoat/Subsystem2/Subsystem3 ==
  CorrienteRuido : Inport
  Constant4 : Constant  Value=1.44
  Constant5 : Constant  Value=5.23
  Gain2 : Gain  Gain=(500/1000000)*41/2
  Gain3 : Gain  Gain=(500/1000000)*41/2
  Gain4 : Gain  Gain=1/1.326
  Sat Cur : Saturate  UpperLimit=3.3  LowerLimit=0
  Sat Cur1 : Saturate  UpperLimit=3.3  LowerLimit=0
  Sum2 : Sum  Inputs=|-+
  Sum3 : Sum  Inputs=|++
  Sum4 : Sum  Inputs=|+-
  I- : Outport
  I+ : Outport  Port=2
  wires:
  Sat Cur/1 -> I-/1
  Sum4/1 -> Gain4/1
  Gain4/1 -> Gain3/1, Gain2/1
  Sat Cur1/1 -> I+/1
  CorrienteRuido/1 -> Sum4/1
  Constant4/1 -> Sum3/2, Sum2/2
  Sum3/1 -> Sat Cur1/1
  Gain2/1 -> Sum2/1
  Sum2/1 -> Sat Cur/1
  Constant5/1 -> Sum4/2
  Gain3/1 -> Sum3/1

== system HIL5DOF_Speedgoat/Subsystem2/Subsystem4 ==
  CorrienteRuido : Inport
  Constant4 : Constant  Value=1.44
  Constant5 : Constant  Value=5.23
  Gain2 : Gain  Gain=(500/1000000)*41/2
  Gain3 : Gain  Gain=(500/1000000)*41/2
  Gain4 : Gain  Gain=1/1.326
  Sat Cur : Saturate  UpperLimit=3.3  LowerLimit=0
  Sat Cur1 : Saturate  UpperLimit=3.3  LowerLimit=0
  Sum2 : Sum  Inputs=|-+
  Sum3 : Sum  Inputs=|++
  Sum4 : Sum  Inputs=|+-
  I- : Outport
  I+ : Outport  Port=2
  wires:
  Sat Cur/1 -> I-/1
  Sum4/1 -> Gain4/1
  Gain4/1 -> Gain3/1, Gain2/1
  Sat Cur1/1 -> I+/1
  CorrienteRuido/1 -> Sum4/1
  Constant4/1 -> Sum3/2, Sum2/2
  Sum3/1 -> Sat Cur1/1
  Gain2/1 -> Sum2/1
  Sum2/1 -> Sat Cur/1
  Constant5/1 -> Sum4/2
  Gain3/1 -> Sum3/1

== system HIL5DOF_Speedgoat/Subsystem2/Subsystem5 ==
  CorrienteRuido : Inport
  Constant4 : Constant  Value=1.44
  Constant5 : Constant  Value=5.23
  Gain2 : Gain  Gain=(500/1000000)*41/2
  Gain3 : Gain  Gain=(500/1000000)*41/2
  Gain4 : Gain  Gain=1/1.326
  Sat Cur : Saturate  UpperLimit=3.3  LowerLimit=0
  Sat Cur1 : Saturate  UpperLimit=3.3  LowerLimit=0
  Sum2 : Sum  Inputs=|-+
  Sum3 : Sum  Inputs=|++
  Sum4 : Sum  Inputs=|+-
  I- : Outport
  I+ : Outport  Port=2
  wires:
  Sat Cur/1 -> I-/1
  Sum4/1 -> Gain4/1
  Gain4/1 -> Gain3/1, Gain2/1
  Sat Cur1/1 -> I+/1
  CorrienteRuido/1 -> Sum4/1
  Constant4/1 -> Sum3/2, Sum2/2
  Sum3/1 -> Sat Cur1/1
  Gain2/1 -> Sum2/1
  Sum2/1 -> Sat Cur/1
  Constant5/1 -> Sum4/2
  Gain3/1 -> Sum3/1

== system HIL5DOF_Speedgoat/Subsystem2/Subsystem6 ==
  CorrienteRuido : Inport
  Constant4 : Constant  Value=1.44
  Constant5 : Constant  Value=5.23
  Gain2 : Gain  Gain=(500/1000000)*41/2
  Gain3 : Gain  Gain=(500/1000000)*41/2
  Gain4 : Gain  Gain=1/1.326
  Sat Cur : Saturate  UpperLimit=3.3  LowerLimit=0
  Sat Cur1 : Saturate  UpperLimit=3.3  LowerLimit=0
  Sum2 : Sum  Inputs=|-+
  Sum3 : Sum  Inputs=|++
  Sum4 : Sum  Inputs=|+-
  I- : Outport
  I+ : Outport  Port=2
  wires:
  Sat Cur/1 -> I-/1
  Sum4/1 -> Gain4/1
  Gain4/1 -> Gain3/1, Gain2/1
  Sat Cur1/1 -> I+/1
  CorrienteRuido/1 -> Sum4/1
  Constant4/1 -> Sum3/2, Sum2/2
  Sum3/1 -> Sat Cur1/1
  Gain2/1 -> Sum2/1
  Sum2/1 -> Sat Cur/1
  Constant5/1 -> Sum4/2
  Gain3/1 -> Sum3/1

== system HIL5DOF_Speedgoat/Subsystem2/Subsystem7 ==
  CorrienteRuido : Inport
  Constant4 : Constant  Value=1.44
  Constant5 : Constant  Value=5.23
  Gain2 : Gain  Gain=(500/1000000)*41/2
  Gain3 : Gain  Gain=(500/1000000)*41/2
  Gain4 : Gain  Gain=1/1.326
  Sat Cur : Saturate  UpperLimit=3.3  LowerLimit=0
  Sat Cur1 : Saturate  UpperLimit=3.3  LowerLimit=0
  Sum2 : Sum  Inputs=|-+
  Sum3 : Sum  Inputs=|++
  Sum4 : Sum  Inputs=|+-
  I- : Outport
  I+ : Outport  Port=2
  wires:
  Sat Cur/1 -> I-/1
  Sum4/1 -> Gain4/1
  Gain4/1 -> Gain3/1, Gain2/1
  Sat Cur1/1 -> I+/1
  CorrienteRuido/1 -> Sum4/1
  Constant4/1 -> Sum3/2, Sum2/2
  Sum3/1 -> Sat Cur1/1
  Gain2/1 -> Sum2/1
  Sum2/1 -> Sat Cur/1
  Constant5/1 -> Sum4/2
  Gain3/1 -> Sum3/1

== system HIL5DOF_Speedgoat/Subsystem2/Subsystem8 ==
  CorrienteRuido : Inport
  Constant4 : Constant  Value=1.44
  Constant5 : Constant  Value=5.23
  Gain2 : Gain  Gain=(500/1000000)*41/2
  Gain3 : Gain  Gain=(500/1000000)*41/2
  Gain4 : Gain  Gain=1/1.326
  Sat Cur : Saturate  UpperLimit=3.3  LowerLimit=0
  Sat Cur1 : Saturate  UpperLimit=3.3  LowerLimit=0
  Sum2 : Sum  Inputs=|-+
  Sum3 : Sum  Inputs=|++
  Sum4 : Sum  Inputs=|+-
  I- : Outport
  I+ : Outport  Port=2
  wires:
  Sat Cur/1 -> I-/1
  Sum4/1 -> Gain4/1
  Gain4/1 -> Gain3/1, Gain2/1
  Sat Cur1/1 -> I+/1
  CorrienteRuido/1 -> Sum4/1
  Constant4/1 -> Sum3/2, Sum2/2
  Sum3/1 -> Sat Cur1/1
  Gain2/1 -> Sum2/1
  Sum2/1 -> Sat Cur/1
  Constant5/1 -> Sum4/2
  Gain3/1 -> Sum3/1

== system HIL5DOF_Speedgoat/Subsystem2/Subsystem9 ==
  CorrienteRuido : Inport
  Constant4 : Constant  Value=1.44
  Constant5 : Constant  Value=5.23
  Gain2 : Gain  Gain=(500/1000000)*41/2
  Gain3 : Gain  Gain=(500/1000000)*41/2
  Gain4 : Gain  Gain=1/1.326
  Sat Cur : Saturate  UpperLimit=3.3  LowerLimit=0
  Sat Cur1 : Saturate  UpperLimit=3.3  LowerLimit=0
  Sum2 : Sum  Inputs=|-+
  Sum3 : Sum  Inputs=|++
  Sum4 : Sum  Inputs=|+-
  I- : Outport
  I+ : Outport  Port=2
  wires:
  Sat Cur/1 -> I-/1
  Sum4/1 -> Gain4/1
  Gain4/1 -> Gain3/1, Gain2/1
  Sat Cur1/1 -> I+/1
  CorrienteRuido/1 -> Sum4/1
  Constant4/1 -> Sum3/2, Sum2/2
  Sum3/1 -> Sat Cur1/1
  Gain2/1 -> Sum2/1
  Sum2/1 -> Sat Cur/1
  Constant5/1 -> Sum4/2
  Gain3/1 -> Sum3/1

== system HIL5DOF_Speedgoat/MODELO ELECTROMAGNÉTICO/MODELO ELECTROMAGNETICO EMS/EMS 1 ==
  Tensión Objetivo : Inport
  Airgap : Inport  Port=2
  2-D Lookup Table1 : Lookup_n-D  BreakpointsForDimension1=ems.Airgap  BreakpointsForDimension2=ems.Current  Table=ems.Force_Horizontal  ExtrapMethod=Clip  InternalRulePriority=Speed  RndMeth=Simplest
      settings: InputPortMap=u0,u1
  CIrcuito RL : Subsystem
  Gain : Gain  Gain=1000
  Modelado Temperatura : Subsystem  Commented=through
  Corriente : Outport
  T [ºC] : Outport  Port=2
  Fuerza Horizontal : Outport  Port=3
  wires:
  2-D Lookup Table1/1 -> Fuerza Horizontal/1
  Modelado Temperatura/1(T [ºC]) -> T [ºC]/1
  Gain/1 -> 2-D Lookup Table1/1
  Airgap/1 -> CIrcuito RL/1(Airgap), Gain/1
  Tensión Objetivo/1 -> CIrcuito RL/2(Tensión Objetivo)
  CIrcuito RL/1(Corriente) -> Corriente/1, Modelado Temperatura/1(I (A)), 2-D Lookup Table1/2

== system HIL5DOF_Speedgoat/MODELO ELECTROMAGNÉTICO/MODELO ELECTROMAGNETICO EMS/EMS 2 ==
  Tensión Objetivo : Inport
  Airgap : Inport  Port=2
  2-D Lookup Table1 : Lookup_n-D  BreakpointsForDimension1=ems.Airgap  BreakpointsForDimension2=ems.Current  Table=ems.Force_Horizontal  ExtrapMethod=Clip  InternalRulePriority=Speed  RndMeth=Simplest
      settings: InputPortMap=u0,u1
  CIrcuito RL : Subsystem
  Gain : Gain  Gain=1000
  Modelado Temperatura : Subsystem  Commented=through
  Corriente : Outport
  T [ºC] : Outport  Port=2
  Fuerza Horizontal : Outport  Port=3
  wires:
  CIrcuito RL/1(Corriente) -> 2-D Lookup Table1/2, Modelado Temperatura/1(I (A)), Corriente/1
  Tensión Objetivo/1 -> CIrcuito RL/2(Tensión Objetivo)
  Airgap/1 -> Gain/1, CIrcuito RL/1(Airgap)
  Gain/1 -> 2-D Lookup Table1/1
  Modelado Temperatura/1(T [ºC]) -> T [ºC]/1
  2-D Lookup Table1/1 -> Fuerza Horizontal/1

== system HIL5DOF_Speedgoat/MODELO ELECTROMAGNÉTICO/MODELO ELECTROMAGNETICO EMS/EMS 3 ==
  Tensión Objetivo : Inport
  Airgap : Inport  Port=2
  2-D Lookup Table1 : Lookup_n-D  BreakpointsForDimension1=ems.Airgap  BreakpointsForDimension2=ems.Current  Table=ems.Force_Horizontal  ExtrapMethod=Clip  InternalRulePriority=Speed  RndMeth=Simplest
      settings: InputPortMap=u0,u1
  CIrcuito RL : Subsystem
  Gain : Gain  Gain=1000
  Modelado Temperatura : Subsystem  Commented=through
  Corriente : Outport
  T [ºC] : Outport  Port=2
  Fuerza Horizontal : Outport  Port=3
  wires:
  2-D Lookup Table1/1 -> Fuerza Horizontal/1
  Modelado Temperatura/1(T [ºC]) -> T [ºC]/1
  Gain/1 -> 2-D Lookup Table1/1
  Airgap/1 -> CIrcuito RL/1(Airgap), Gain/1
  Tensión Objetivo/1 -> CIrcuito RL/2(Tensión Objetivo)
  CIrcuito RL/1(Corriente) -> Corriente/1, Modelado Temperatura/1(I (A)), 2-D Lookup Table1/2

== system HIL5DOF_Speedgoat/MODELO ELECTROMAGNÉTICO/MODELO ELECTROMAGNETICO EMS/EMS 4 ==
  Tensión Objetivo : Inport
  Airgap : Inport  Port=2
  2-D Lookup Table1 : Lookup_n-D  BreakpointsForDimension1=ems.Airgap  BreakpointsForDimension2=ems.Current  Table=ems.Force_Horizontal  ExtrapMethod=Clip  InternalRulePriority=Speed  RndMeth=Simplest
      settings: InputPortMap=u0,u1
  CIrcuito RL : Subsystem
  Gain : Gain  Gain=1000
  Modelado Temperatura : Subsystem  Commented=through
  Corriente : Outport
  T [ºC] : Outport  Port=2
  Fuerza Horizontal : Outport  Port=3
  wires:
  CIrcuito RL/1(Corriente) -> 2-D Lookup Table1/2, Modelado Temperatura/1(I (A)), Corriente/1
  Tensión Objetivo/1 -> CIrcuito RL/2(Tensión Objetivo)
  Airgap/1 -> Gain/1, CIrcuito RL/1(Airgap)
  Gain/1 -> 2-D Lookup Table1/1
  Modelado Temperatura/1(T [ºC]) -> T [ºC]/1
  2-D Lookup Table1/1 -> Fuerza Horizontal/1

== system HIL5DOF_Speedgoat/MODELO ELECTROMAGNÉTICO/MODELO ELECTROMAGNETICO EMS/EMS 5 ==
  Tensión Objetivo : Inport
  Airgap : Inport  Port=2
  2-D Lookup Table1 : Lookup_n-D  BreakpointsForDimension1=ems.Airgap  BreakpointsForDimension2=ems.Current  Table=ems.Force_Horizontal  ExtrapMethod=Clip  InternalRulePriority=Speed  RndMeth=Simplest
      settings: InputPortMap=u0,u1
  CIrcuito RL : Subsystem
  Gain : Gain  Gain=1000
  Modelado Temperatura : Subsystem  Commented=through
  Corriente : Outport
  T [ºC] : Outport  Port=2
  Fuerza Horizontal : Outport  Port=3
  wires:
  2-D Lookup Table1/1 -> Fuerza Horizontal/1
  Modelado Temperatura/1(T [ºC]) -> T [ºC]/1
  Gain/1 -> 2-D Lookup Table1/1
  Airgap/1 -> CIrcuito RL/1(Airgap), Gain/1
  Tensión Objetivo/1 -> CIrcuito RL/2(Tensión Objetivo)
  CIrcuito RL/1(Corriente) -> Corriente/1, Modelado Temperatura/1(I (A)), 2-D Lookup Table1/2
